simulink model "msbr_pke_stat"  (R2015b)
settings: Solver=ode45  StartTime=0.0  StopTime=20000  RelTol=1e-3
values from neighbouring files (symbols this model uses):
  beta = [2.290E-04, 8.320E-04, 7.100E-04, 8.520E-04, 1.710E-04, 1.020E-04]    [Parameters_Core_PHE.m]    (also in Parameters_Core_PHE_FEHE.m; Parameters_MSBR.m; Parameters_MSBR_Brayton.m; Parameters_MSBR_new_nodal.m)
  beta_t = sum(beta)    [Parameters_Core_PHE.m]    (also in Parameters_Core_PHE_FEHE.m; Parameters_MSBR.m; Parameters_MSBR_Brayton.m; Parameters_MSBR_new_nodal.m)
  C0 = lam.\beta/Lam    [parameters_msbr_pke_stat.m]
  Lam = 3.300E-04    (= 0.00033)    [Parameters_Core_PHE.m]    (also in Parameters_Core_PHE_FEHE.m; Parameters_MSBR.m; Parameters_MSBR_Brayton.m; Parameters_MSBR_new_nodal.m)
  lam = [0.0126,0.0337,0.139,0.325,1.13,2.50]'    [PKE_general.m]    (also in Parameters_Core_PHE.m = [1.260E-02, 3.370E-02, 1.390E-01, 3.250E-01, 1.130E+00, 2.50; Parameters_Core_PHE_FEHE.m = [1.260E-02, 3.370E-02, 1.390E-01, 3.250E-01, 1.130E+00, 2.50; Parameters_MSBR.m = [1.260E-02, 3.370E-02, 1.390E-01, 3.250E-01, 1.130E+00, 2.50; Parameters_MSBR_Brayton.m = [1.260E-02, 3.370E-02, 1.390E-01, 3.250E-01, 1.130E+00, 2.50)
  n_frac0 = 1    [Parameters_Core_PHE.m]    (also in Parameters_Core_PHE_FEHE.m; Parameters_MSBR.m; Parameters_MSBR_Brayton.m; Parameters_MSBR_new_nodal.m)
settings Model: Creator=mlish  LastModifiedBy=mlish
settings DataIOCC: LimitDataPoints=off

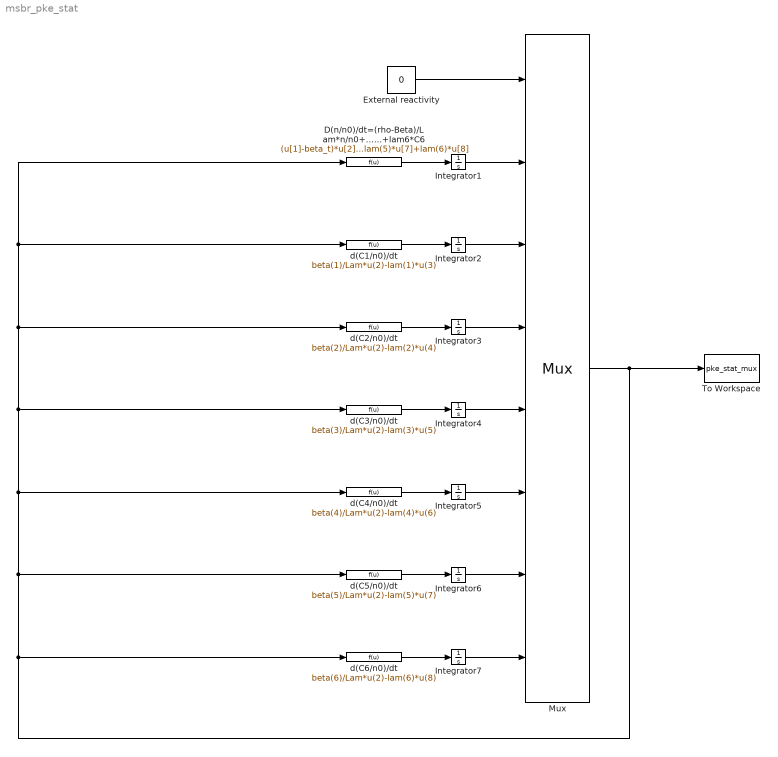
== system msbr_pke_stat ==
  D(n/n0)/dt=(rho-Beta)/Lam*n/n0+lam1*C1+...+lam6*C6 : Fcn  Expr=(u[1]-beta_t)*u[2]/Lam+lam(1)*u[3]+lam(2)*u[4]+lam(3)*u[5]+lam(4)*u[6]+lam(5)*u[7]+lam(6)*u[8]
  External reactivity : Constant  Value=0
  Integrator1 : Integrator  InitialCondition=n_frac0
  Integrator2 : Integrator  InitialCondition=C0(1)
  Integrator3 : Integrator  InitialCondition=C0(2)
  Integrator4 : Integrator  InitialCondition=C0(3)
  Integrator5 : Integrator  InitialCondition=C0(4)
  Integrator6 : Integrator  InitialCondition=C0(5)
  Integrator7 : Integrator  InitialCondition=C0(6)
  Mux : Mux  Inputs=8
      settings: DisplayOption=signals
  To Workspace : ToWorkspace  VariableName=pke_stat_mux  SampleTime=-1
  d(C1/n0)/dt : Fcn  Expr=beta(1)/Lam*u(2)-lam(1)*u(3)
  d(C2/n0)/dt : Fcn  Expr=beta(2)/Lam*u(2)-lam(2)*u(4)
  d(C3/n0)/dt : Fcn  Expr=beta(3)/Lam*u(2)-lam(3)*u(5)
  d(C4/n0)/dt : Fcn  Expr=beta(4)/Lam*u(2)-lam(4)*u(6)
  d(C5/n0)/dt : Fcn  Expr=beta(5)/Lam*u(2)-lam(5)*u(7)
  d(C6/n0)/dt : Fcn  Expr=beta(6)/Lam*u(2)-lam(6)*u(8)
  wires:
  Mux/1 -> d(C6/n0)/dt/1, d(C5/n0)/dt/1, d(C4/n0)/dt/1, d(C3/n0)/dt/1, d(C2/n0)/dt/1, D(n/n0)/dt=(rho-Beta)/Lam*n/n0+lam1*C1+...+lam6*C6/1, d(C1/n0)/dt/1, To Workspace/1
  D(n/n0)/dt=(rho-Beta)/Lam*n/n0+lam1*C1+...+lam6*C6/1 -> Integrator1/1
  d(C1/n0)/dt/1 -> Integrator2/1
  d(C2/n0)/dt/1 -> Integrator3/1
  d(C3/n0)/dt/1 -> Integrator4/1
  d(C4/n0)/dt/1 -> Integrator5/1
  d(C5/n0)/dt/1 -> Integrator6/1
  d(C6/n0)/dt/1 -> Integrator7/1
  External reactivity/1 -> Mux/1
  Integrator1/1 -> Mux/2
  Integrator2/1 -> Mux/3
  Integrator3/1 -> Mux/4
  Integrator4/1 -> Mux/5
  Integrator5/1 -> Mux/6
  Integrator6/1 -> Mux/7
  Integrator7/1 -> Mux/8
